simulink model "seguidor_completo_feed_wind_smith"  (R2019a)
settings: Solver=VariableStepAuto  StartTime=0.0  StopTime=600  RelTol=1e-3
values from neighbouring files (symbols this model uses):
  hdis2 = hdis2'    [programa_seguidor.m]
  ki = ka(1:end,m+1:end)    [programa_seguidor.m]
  kidis2 = ktdis2(:,m+1:end)    [programa_seguidor.m]
  kp = ka(1:end,1:m)    [programa_seguidor.m]
  kpdis2 = ktdis2(:,1:m)    [programa_seguidor.m]
  tm2 = 10    [programa_seguidor.m]
undefined symbols (not defined in the file or in its folder): A, A2, adis2, B, B2, bdis2, C, C2, cdis2
settings Model: Creator=Alejoxbg  LastModifiedBy=Alejoxbg

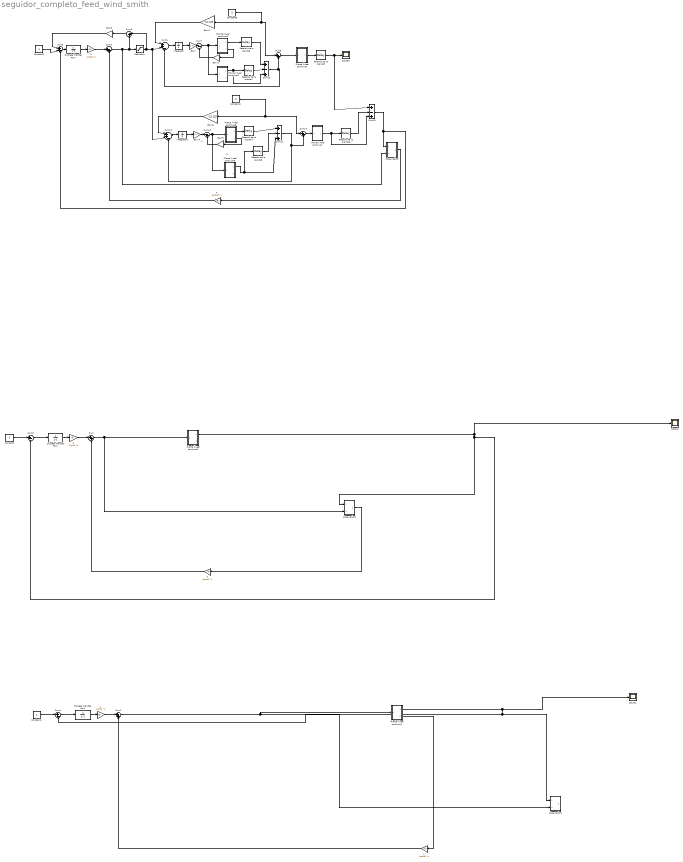
== system seguidor_completo_feed_wind_smith ==
  note: -ki
  note: -kp
  " 1" : Gain  Gain=-kpdis2  Multiplication=Matrix(K*u) (u vector)  SampleTime=tm2
  " 2" : Gain  Gain=-kpdis2  Multiplication=Matrix(K*u) (u vector)  SampleTime=tm2
  " 4" : Gain  Gain=-kpdis2  Multiplication=Matrix(K*u) (u vector)  SampleTime=tm2
  " 1" : Gain  Gain=-kidis2  Multiplication=Matrix(K*u) (u vector)  SampleTime=tm2
  " 2" : Gain  Gain=-kidis2  Multiplication=Matrix(K*u) (u vector)  SampleTime=tm2
  " 3" : Gain  Gain=-kidis2  Multiplication=Matrix(K*u) (u vector)  SampleTime=tm2
  Constant : Constant
  Constant1 : Constant
  Constant2 : Constant
  Constant3 : Constant  Value=2
  Constant4 : Constant  Value=2
  Discrete Transfer Fcn1 : DiscreteTransferFcn  Numerator=[1 0]  Denominator=[1 -1]  SampleTime=tm2  a0EqualsOne=on
  Discrete Transfer Fcn2 : DiscreteTransferFcn  Numerator=[1 0]  Denominator=[1 -1]  SampleTime=tm2  a0EqualsOne=on
  Discrete Transfer Fcn4 : DiscreteTransferFcn  Numerator=[1 0]  Denominator=[1 -1]  SampleTime=tm2  a0EqualsOne=on
  Gain : Gain  Gain=ki  Multiplication=Matrix(K*u) (u vector)
  Gain1 : Gain  Gain=kp  Multiplication=Matrix(K*u) (u vector)
  Gain2 : Gain  Gain=-1/1.125
  Gain3 : Gain  Gain=0.1  Multiplication=Matrix(K*u) (u vector)
  Gain4 : Gain  Gain=ki  Multiplication=Matrix(K*u) (u vector)
  Gain5 : Gain  Gain=kp  Multiplication=Matrix(K*u) (u vector)
  Gain6 : Gain  Gain=-1/1.125
  Integrator : Integrator
  Integrator1 : Integrator
  Planta lineal continua1 : Subsystem
  Planta lineal continua2 : Subsystem
  Planta lineal continua3 : Subsystem
  Planta lineal continua4 : Subsystem
  Planta lineal continua5 : Subsystem
  Planta lineal continua6 : Subsystem
  Planta lineal continua7 : Subsystem
  Planta lineal continua8 : Subsystem
  Retardo de la planta{1..6} (6 alike) : TransportDelay  DelayTime=10
  Saturation : Saturate  UpperLimit=5  LowerLimit=-5  ZeroCross=off
  Scope1 : Scope
  Scope3 : Scope
  Scope7 : Scope
  Sum{,1..2,8,14} (5 alike) : Sum  Inputs=|++
  Sum10 : Sum  Inputs=|+-+
  Sum11 : Sum  Inputs=|+-+
  Sum12 : Sum  Inputs=|++-
  Sum13 : Sum  Inputs=|--
  Sum15 : Sum  Inputs=|+-+
  Sum3 : Sum  Inputs=|+-
  Sum4 : Sum  Inputs=|+-
  Sum5 : Sum  Inputs=|++-
  Sum6 : Sum  Inputs=|++-
  Sum7 : Sum  Inputs=|--
  Sum9 : Sum  Inputs=|-+
  observador1 : Subsystem
  observador2 : Subsystem
  observador3 : Subsystem
  wires:
  Planta lineal continua2/1(y) -> Sum3/2, observador2/1(y), Scope7/1
  Sum/1 -> Planta lineal continua2/1(u), observador2/2(u)
  Discrete Transfer Fcn1/1 -> " 2"/1
  " 2"/1 -> Sum/1
  observador2/1(xgorro) -> " 2"/1
  " 2"/1 -> Sum/2
  Sum3/1 -> Discrete Transfer Fcn1/1
  Constant/1 -> Sum3/1
  Discrete Transfer Fcn2/1 -> " 1"/1
  Planta lineal continua1/1(y) -> observador1/1(y), Sum4/2, Scope1/1
  Constant1/1 -> Sum4/1
  " 1"/1 -> Sum1/1
  " 1"/1 -> Sum1/2
  Sum4/1 -> Discrete Transfer Fcn2/1
  Sum1/1 -> Planta lineal continua1/1(u), observador1/2(u)
  Planta lineal continua1/2("X ") -> " 1"/1
  " 4"/1 -> Sum2/2
  observador3/1(xgorro) -> " 4"/1
  Constant2/1 -> Sum5/2
  " 3"/1 -> Sum2/1
  Sum5/1 -> Discrete Transfer Fcn4/1
  Discrete Transfer Fcn4/1 -> " 3"/1
  Sum6/1 -> Integrator/1
  Gain1/1 -> Sum7/2
  Integrator/1 -> Gain/1
  Planta lineal continua3/2(x) -> Gain1/1
  Sum2/1 -> observador3/2(u), Sum9/2, Saturation/1
  Gain/1 -> Sum7/1
  Gain2/1 -> Sum6/1
  Constant3/1 -> Sum8/1, Gain2/1
  Sum8/1 -> Planta lineal continua4/1(u)
  Sum7/1 -> Planta lineal continua3/1(u), Planta lineal continua5/1(u)
  Sum9/1 -> Gain3/1
  Gain3/1 -> Sum5/1
  Planta lineal continua5/1(y) -> Sum10/3, Retardo de la planta1/1
  Planta lineal continua3/1(y) -> Retardo de la planta2/1
  Retardo de la planta2/1 -> Sum10/1
  Sum10/1 -> Sum6/3, Sum8/2
  Retardo de la planta1/1 -> Sum10/2
  Sum11/1 -> Sum12/3, Sum14/2
  Retardo de la planta3/1 -> Sum11/2
  Constant4/1 -> Sum14/1, Gain6/1
  Gain6/1 -> Sum12/1
  Saturation/1 -> Sum9/1, Sum12/2, Sum6/2
  Sum13/1 -> Planta lineal continua8/1(u), Planta lineal continua6/1(u)
  Gain4/1 -> Sum13/1
  Gain5/1 -> Sum13/2
  Sum12/1 -> Integrator1/1
  Planta lineal continua6/2(x) -> Gain5/1
  Retardo de la planta4/1 -> Sum11/1
  Integrator1/1 -> Gain4/1
  Planta lineal continua6/1(y) -> Retardo de la planta4/1
  Planta lineal continua8/1(y) -> Sum11/3, Retardo de la planta3/1
  Sum14/1 -> Planta lineal continua7/1(u)
  Planta lineal continua4/1(y) -> Retardo de la planta5/1
  Planta lineal continua7/1(y) -> Sum15/3, Retardo de la planta6/1
  Retardo de la planta5/1 -> Scope3/1, Sum15/1
  Retardo de la planta6/1 -> Sum15/2
  Sum15/1 -> Sum5/3, observador3/1(y)

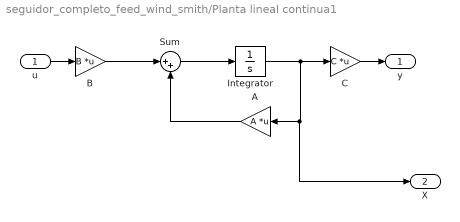
== system seguidor_completo_feed_wind_smith/Planta lineal continua1 ==
  u : Inport
  A : Gain  Gain=A  Multiplication=Matrix(K*u) (u vector)
  B : Gain  Gain=B  Multiplication=Matrix(K*u) (u vector)
  C : Gain  Gain=C  Multiplication=Matrix(K*u) (u vector)
  Integrator : Integrator
  Sum : Sum  Inputs=|++
  y : Outport
  "X " : Outport  Port=2
  wires:
  C/1 -> y/1
  u/1 -> B/1
  Integrator/1 -> "X "/1, A/1, C/1
  A/1 -> Sum/2
  Sum/1 -> Integrator/1
  B/1 -> Sum/1

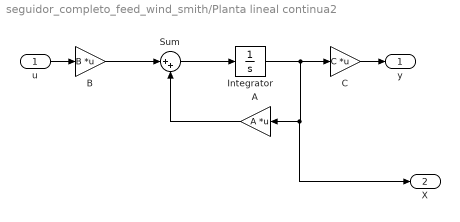
== system seguidor_completo_feed_wind_smith/Planta lineal continua2 ==
  u : Inport
  A : Gain  Gain=A  Multiplication=Matrix(K*u) (u vector)
  B : Gain  Gain=B  Multiplication=Matrix(K*u) (u vector)
  C : Gain  Gain=C  Multiplication=Matrix(K*u) (u vector)
  Integrator : Integrator
  Sum : Sum  Inputs=|++
  y : Outport
  "X " : Outport  Port=2
  wires:
  C/1 -> y/1
  u/1 -> B/1
  Integrator/1 -> "X "/1, A/1, C/1
  A/1 -> Sum/2
  Sum/1 -> Integrator/1
  B/1 -> Sum/1

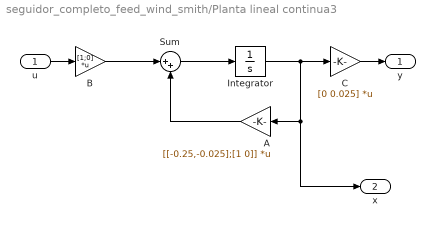
== system seguidor_completo_feed_wind_smith/Planta lineal continua3 ==
  u : Inport
  A : Gain  Gain=[[-0.25,-0.025];[1 0]]  Multiplication=Matrix(K*u) (u vector)
  B : Gain  Gain=[1;0]  Multiplication=Matrix(K*u) (u vector)
  C : Gain  Gain=[0 0.025]  Multiplication=Matrix(K*u) (u vector)
  Integrator : Integrator
  Sum : Sum  Inputs=|++
  y : Outport
  x : Outport  Port=2
  wires:
  C/1 -> y/1
  u/1 -> B/1
  Integrator/1 -> x/1, A/1, C/1
  A/1 -> Sum/2
  Sum/1 -> Integrator/1
  B/1 -> Sum/1

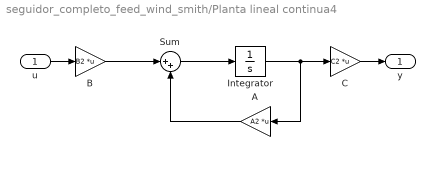
== system seguidor_completo_feed_wind_smith/Planta lineal continua4 ==
  u : Inport
  A : Gain  Gain=A2  Multiplication=Matrix(K*u) (u vector)
  B : Gain  Gain=B2  Multiplication=Matrix(K*u) (u vector)
  C : Gain  Gain=C2  Multiplication=Matrix(K*u) (u vector)
  Integrator : Integrator
  Sum : Sum  Inputs=|++
  y : Outport
  wires:
  C/1 -> y/1
  u/1 -> B/1
  Integrator/1 -> A/1, C/1
  A/1 -> Sum/2
  Sum/1 -> Integrator/1
  B/1 -> Sum/1

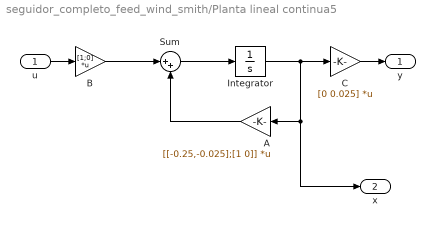
== system seguidor_completo_feed_wind_smith/Planta lineal continua5 ==
  u : Inport
  A : Gain  Gain=[[-0.25,-0.025];[1 0]]  Multiplication=Matrix(K*u) (u vector)
  B : Gain  Gain=[1;0]  Multiplication=Matrix(K*u) (u vector)
  C : Gain  Gain=[0 0.025]  Multiplication=Matrix(K*u) (u vector)
  Integrator : Integrator
  Sum : Sum  Inputs=|++
  y : Outport
  x : Outport  Port=2
  wires:
  C/1 -> y/1
  u/1 -> B/1
  Integrator/1 -> x/1, A/1, C/1
  A/1 -> Sum/2
  Sum/1 -> Integrator/1
  B/1 -> Sum/1

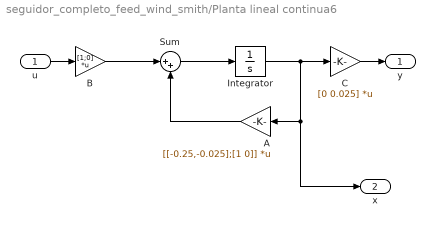
== system seguidor_completo_feed_wind_smith/Planta lineal continua6 ==
  u : Inport
  A : Gain  Gain=[[-0.25,-0.025];[1 0]]  Multiplication=Matrix(K*u) (u vector)
  B : Gain  Gain=[1;0]  Multiplication=Matrix(K*u) (u vector)
  C : Gain  Gain=[0 0.025]  Multiplication=Matrix(K*u) (u vector)
  Integrator : Integrator
  Sum : Sum  Inputs=|++
  y : Outport
  x : Outport  Port=2
  wires:
  C/1 -> y/1
  u/1 -> B/1
  Integrator/1 -> x/1, A/1, C/1
  A/1 -> Sum/2
  Sum/1 -> Integrator/1
  B/1 -> Sum/1

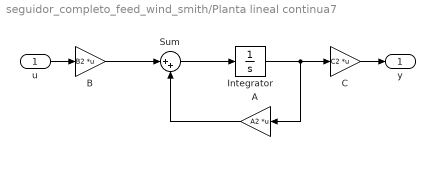
== system seguidor_completo_feed_wind_smith/Planta lineal continua7 ==
  u : Inport
  A : Gain  Gain=A2  Multiplication=Matrix(K*u) (u vector)
  B : Gain  Gain=B2  Multiplication=Matrix(K*u) (u vector)
  C : Gain  Gain=C2  Multiplication=Matrix(K*u) (u vector)
  Integrator : Integrator
  Sum : Sum  Inputs=|++
  y : Outport
  wires:
  C/1 -> y/1
  u/1 -> B/1
  Integrator/1 -> A/1, C/1
  A/1 -> Sum/2
  Sum/1 -> Integrator/1
  B/1 -> Sum/1

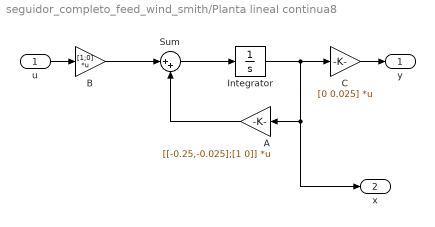
== system seguidor_completo_feed_wind_smith/Planta lineal continua8 ==
  u : Inport
  A : Gain  Gain=[[-0.25,-0.025];[1 0]]  Multiplication=Matrix(K*u) (u vector)
  B : Gain  Gain=[1;0]  Multiplication=Matrix(K*u) (u vector)
  C : Gain  Gain=[0 0.025]  Multiplication=Matrix(K*u) (u vector)
  Integrator : Integrator
  Sum : Sum  Inputs=|++
  y : Outport
  x : Outport  Port=2
  wires:
  C/1 -> y/1
  u/1 -> B/1
  Integrator/1 -> x/1, A/1, C/1
  A/1 -> Sum/2
  Sum/1 -> Integrator/1
  B/1 -> Sum/1

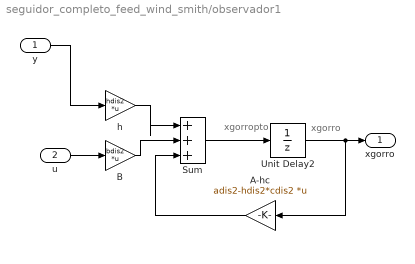
== system seguidor_completo_feed_wind_smith/observador1 ==
  note: xgorro
  note: xgorropto
  y : Inport
  u : Inport  Port=2
  A-hc : Gain  Gain=adis2-hdis2*cdis2  Multiplication=Matrix(K*u) (u vector)
  B : Gain  Gain=bdis2  Multiplication=Matrix(K*u) (u vector)
  Sum : Sum  Inputs=|+++
  Unit Delay2 : UnitDelay  SampleTime=tm2  HasFrameUpgradeWarning=on
  h : Gain  Gain=hdis2  Multiplication=Matrix(K*u) (u vector)
  xgorro : Outport
  wires:
  u/1 -> B/1
  h/1 -> Sum/1
  B/1 -> Sum/2
  A-hc/1 -> Sum/3
  Unit Delay2/1 -> xgorro/1, A-hc/1
  Sum/1 -> Unit Delay2/1
  y/1 -> h/1

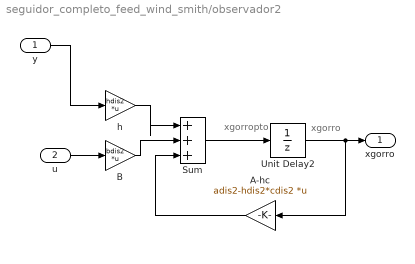
== system seguidor_completo_feed_wind_smith/observador2 ==
  note: xgorro
  note: xgorropto
  y : Inport
  u : Inport  Port=2
  A-hc : Gain  Gain=adis2-hdis2*cdis2  Multiplication=Matrix(K*u) (u vector)
  B : Gain  Gain=bdis2  Multiplication=Matrix(K*u) (u vector)
  Sum : Sum  Inputs=|+++
  Unit Delay2 : UnitDelay  SampleTime=tm2  HasFrameUpgradeWarning=on
  h : Gain  Gain=hdis2  Multiplication=Matrix(K*u) (u vector)
  xgorro : Outport
  wires:
  u/1 -> B/1
  h/1 -> Sum/1
  B/1 -> Sum/2
  A-hc/1 -> Sum/3
  Unit Delay2/1 -> xgorro/1, A-hc/1
  Sum/1 -> Unit Delay2/1
  y/1 -> h/1

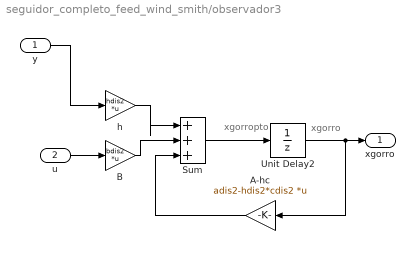
== system seguidor_completo_feed_wind_smith/observador3 ==
  note: xgorro
  note: xgorropto
  y : Inport
  u : Inport  Port=2
  A-hc : Gain  Gain=adis2-hdis2*cdis2  Multiplication=Matrix(K*u) (u vector)
  B : Gain  Gain=bdis2  Multiplication=Matrix(K*u) (u vector)
  Sum : Sum  Inputs=|+++
  Unit Delay2 : UnitDelay  SampleTime=tm2  HasFrameUpgradeWarning=on
  h : Gain  Gain=hdis2  Multiplication=Matrix(K*u) (u vector)
  xgorro : Outport
  wires:
  u/1 -> B/1
  h/1 -> Sum/1
  B/1 -> Sum/2
  A-hc/1 -> Sum/3
  Unit Delay2/1 -> xgorro/1, A-hc/1
  Sum/1 -> Unit Delay2/1
  y/1 -> h/1
